simulink model "furuta_pendulum_response"  (R2016a)
settings: Solver=VariableStepAuto  StartTime=0.0  StopTime=10.0  MaxStep=1e-3  RelTol=1e-3
settings Model: Creator=mgreiff  LastModifiedBy=mgreiff

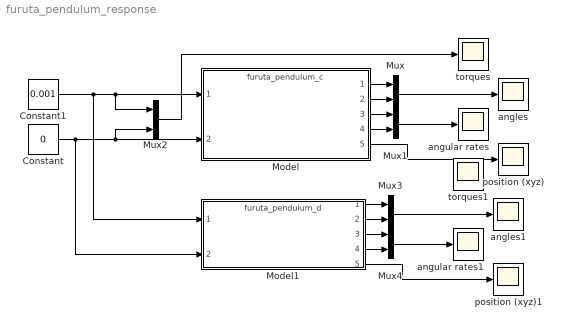
== system furuta_pendulum_response ==
  Constant : Constant  Value=0
  Constant1 : Constant  Value=0.001
  Model : ModelReference  ModelNameDialog=furuta_pendulum_c.slx  SimulationMode=Normal  ModelReferenceVersion=1.33
  Model1 : ModelReference  ModelNameDialog=furuta_pendulum_d.slx  SimulationMode=Normal  ModelReferenceVersion=1.44
  Mux{,1..4} (5 alike) : Mux  Inputs=2
  angles : Scope
  angles1 : Scope
  angular rates : Scope
  angular rates1 : Scope
  position (xyz) : Scope
  position (xyz)1 : Scope
  torques : Scope
  torques1 : Scope
  wires:
  Model/1 -> Mux/1
  Model/3 -> Mux1/1
  Model/4 -> Mux1/2
  Mux1/1 -> angular rates/1
  Model/2 -> Mux/2
  Mux/1 -> angles/1
  Mux2/1 -> torques/1
  Constant1/1 -> Model1/1, Mux2/1, Model/1
  Constant/1 -> Model1/2, Mux2/2, Model/2
  Model/5 -> position (xyz)/1
  Model1/1 -> Mux3/1
  Model1/3 -> Mux4/1
  Model1/4 -> Mux4/2
  Mux4/1 -> angular rates1/1
  Model1/2 -> Mux3/2
  Mux3/1 -> angles1/1
  Model1/5 -> position (xyz)1/1
